simulink model "ABFTSMC"  (R2021b)
settings: Solver=VariableStepAuto  StartTime=0.0  StopTime=70  RelTol=1e-3
values from neighbouring files (symbols this model uses):
  a1 = (Iyy-Izz)/Ixx    [ABFTSMC_script.m]    (also in parameters_ABFTSMC.m = -1.00067938333)
  a10 = -kdy/m    [ABFTSMC_script.m]    (also in parameters_ABFTSMC.m = -0.00114547325103)
  a11 = -kdz/m    [ABFTSMC_script.m]    (also in parameters_ABFTSMC.m = -0.00114547325103)
  a3 = -kax/Ixx    [ABFTSMC_script.m]    (also in parameters_ABFTSMC.m = -0.145466422785)
  a4 = (Izz-Ixx)/Iyy    [ABFTSMC_script.m]    (also in parameters_ABFTSMC.m = 1.00067938333)
  a6 = -kay/Iyy    [ABFTSMC_script.m]    (also in parameters_ABFTSMC.m = -0.145466422785)
  a7 = (Ixx-Iyy)/Izz    [ABFTSMC_script.m]    (also in parameters_ABFTSMC.m = 0)
  a8 = -kaz/Izz    [ABFTSMC_script.m]    (also in parameters_ABFTSMC.m = -0.072708512917)
  a9 = -kdx/m    [ABFTSMC_script.m]    (also in parameters_ABFTSMC.m = -0.00114547325103)
  alpha_phi = 10    [ABFTSMC_script.m]    (also in parameters_ABFTSMC.m = 9.3414)
  alpha_si = 9.3414    [parameters_ABFTSMC.m]
  alpha_theta = alpha_phi    (= 10)    [ABFTSMC_script.m]    (also in parameters_ABFTSMC.m = 9.3414)
  b1 = 1/Ixx    [ABFTSMC_script.m]    (also in parameters_ABFTSMC.m = 39.1951920564)
  b2 = 1/Iyy    [ABFTSMC_script.m]    (also in parameters_ABFTSMC.m = 39.1951920564)
  b3 = 1/Izz    [ABFTSMC_script.m]    (also in parameters_ABFTSMC.m = 130.606274325)
  beta_phi = 0.2146    [ABFTSMC_script.m]    (also in parameters_ABFTSMC.m)
  beta_si = 0.2146    [parameters_ABFTSMC.m]
  beta_theta = beta_phi    (= 0.2146)    [ABFTSMC_script.m]    (also in parameters_ABFTSMC.m)
  c_phi = 0.01    [ABFTSMC_script.m]    (also in parameters_ABFTSMC.m = 0.0527)
  c_si = 0.0527    [parameters_ABFTSMC.m]
  c_theta = c_phi    (= 0.01)    [ABFTSMC_script.m]    (also in parameters_ABFTSMC.m = 0.0527)
  cd = Parameters.cd    [ABFTSMC_script.m]    (also in parameters_ABFTSMC.m = 0.03232)
  cx1 = 0.8    [ABFTSMC_script.m]    (also in parameters_ABFTSMC.m = 3.227)
  cy1 = 4    [ABFTSMC_script.m]    (also in parameters_ABFTSMC.m = 3.227)
  cz1 = 5    [ABFTSMC_script.m]    (also in parameters_ABFTSMC.m = 3.227)
  g = Parameters.g    [ABFTSMC_script.m]    (also in parameters_ABFTSMC.m = 9.81)
  gama11 = 0.1    [parameters_ABFTSMC.m]
  gama7 = 0.1    [parameters_ABFTSMC.m]
  gama9 = 0.1    [parameters_ABFTSMC.m]
  gama_phi = 17.4513    [parameters_ABFTSMC.m]
  gama_si = 17.4513    [parameters_ABFTSMC.m]
  gama_theta = 17.4513    [parameters_ABFTSMC.m]
  Ir = Parameters.Ir    [ABFTSMC_script.m]    (also in parameters_ABFTSMC.m = 2.8385e-05)
  Ixx = Parameters.Ixx    [ABFTSMC_script.m]    (also in parameters_ABFTSMC.m = 0.003827)
  Iyy = Parameters.Iyy    [ABFTSMC_script.m]    (also in parameters_ABFTSMC.m = 0.003827)
  kp = Parameters.kp    [ABFTSMC_script.m]    (also in parameters_ABFTSMC.m = 0.0029842)
  m = Parameters.m    [ABFTSMC_script.m]    (also in parameters_ABFTSMC.m = 0.486)
  mu = [mu_phi mu_theta mu_say]'    [ABFTSMC_script.m]    (also in parameters_ABFTSMC.m = 0.01*ones(3,1))
  p_phi = 3    [ABFTSMC_script.m]    (also in parameters_ABFTSMC.m = 2.4429)
  p_si = 2.4429    [parameters_ABFTSMC.m]
  p_theta = p_phi    (= 3)    [ABFTSMC_script.m]    (also in parameters_ABFTSMC.m = 2.4429)
  q_phi = 5    [ABFTSMC_script.m]    (also in parameters_ABFTSMC.m = 4.3864)
  q_si = 4.3864    [parameters_ABFTSMC.m]
  q_theta = q_phi    (= 5)    [ABFTSMC_script.m]    (also in parameters_ABFTSMC.m = 4.3864)
undefined symbols (not defined in the file or in its folder): magnitude
libraries: dspinverses x1
settings Model: Creator=alikh  LastModifiedBy=alikh

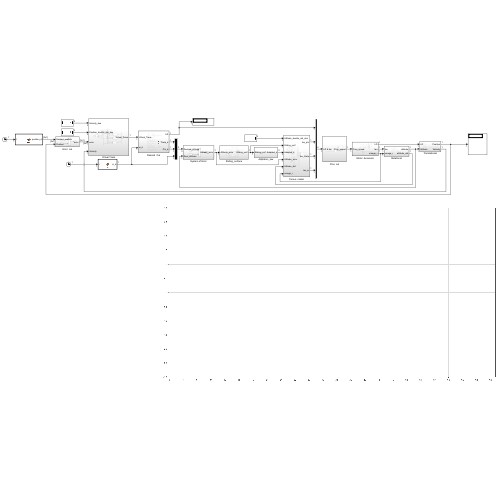
[thumbnail: Simulink's stored preview of the top-level diagram]
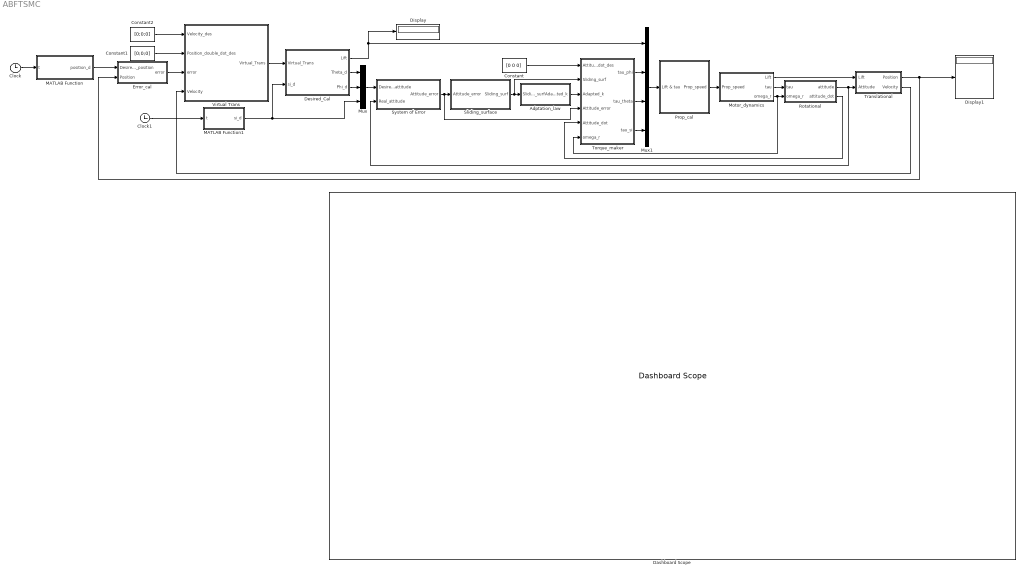
== system ABFTSMC ==
  Adptation_law : Subsystem
  Clock : Clock
  Clock1 : Clock
  Constant : Constant  Value=[0 0 0]
  Constant1 : Constant  Value=[0;0;0]
  Constant2 : Constant  Value=[0;0;0]
  Dashboard Scope : DashboardScope
  Desired_Cal : Subsystem
  Display : Display
  Display1 : Display
  Error_cal : Subsystem
  MATLAB Function : MATLAB Function  TreatAsAtomicUnit=on
  MATLAB Function1 : MATLAB Function  TreatAsAtomicUnit=on
  Motor_dynamics : Subsystem
  Mux : Mux  Inputs=3
  Mux1 : Mux
  Prop_cal : Subsystem
  Rotational : Subsystem
  Sliding_surface : Subsystem
  System of Error : Subsystem
  Torque_maker : Subsystem
  Translational : Subsystem
  Virtual Trans : Subsystem
  wires:
  Virtual Trans/1(Virtual_Trans) -> Desired_Cal/1(Virtual_Trans)
  MATLAB Function1/1(si_d) -> Desired_Cal/2(si_d), Mux/3
  Desired_Cal/2(Theta_d) -> Mux/1
  Desired_Cal/3(Phi_d) -> Mux/2
  Mux/1 -> System of Error/1(Desired_attitude)
  Desired_Cal/1(Lift) -> Display/1, Mux1/1
  System of Error/1(Attitude_error) -> Sliding_surface/1(Attitude_error), Torque_maker/4(Attitude_error)
  Sliding_surface/1(Sliding_surf) -> Torque_maker/2(Sliding_surf), Adptation_law/1(Sliding_surf)
  Adptation_law/1(Adapted_k) -> Torque_maker/3(Adapted_k)
  Torque_maker/1(tau_phi) -> Mux1/2
  Torque_maker/2(tau_theta) -> Mux1/3
  Torque_maker/3(tau_si) -> Mux1/4
  Mux1/1 -> Prop_cal/1(Lift & tau)
  Prop_cal/1(Prop_speed) -> Motor_dynamics/1(Prop_speed)
  Motor_dynamics/1(Lift) -> Translational/1(Lift)
  Motor_dynamics/2(tau) -> Rotational/1(tau)
  Motor_dynamics/3(omega_r) -> Torque_maker/6(omega_r), Rotational/2(omega_r)
  Rotational/2(attitude_dot) -> Torque_maker/5(Attitude_dot)
  Rotational/1(attitude) -> System of Error/2(Real_attitude), Translational/2(Attitude)
  Translational/2(Velocity) -> Virtual Trans/4(Velocity)
  Translational/1(Position) -> Error_cal/2(Position), Display1/1
  Error_cal/1(error) -> Virtual Trans/3(error)
  Constant/1 -> Torque_maker/1(Attitude_double_dot_des)
  Constant1/1 -> Virtual Trans/2(Position_double_dot_des)
  MATLAB Function/1(position_d) -> Error_cal/1(Desired_position)
  Clock/1 -> MATLAB Function/1(t)
  Clock1/1 -> MATLAB Function1/1(t)
  Constant2/1 -> Virtual Trans/1(Velocity_des)

== system ABFTSMC/Adptation_law ==
  Sliding_surf : Inport
  Abs : Abs
  Gain : Gain  Gain=[gama_phi gama_theta gama_si]'
  Integrator : Integrator
  Adapted_k : Outport
  wires:
  Gain/1 -> Integrator/1
  Sliding_surf/1 -> Abs/1
  Integrator/1 -> Adapted_k/1
  Abs/1 -> Gain/1

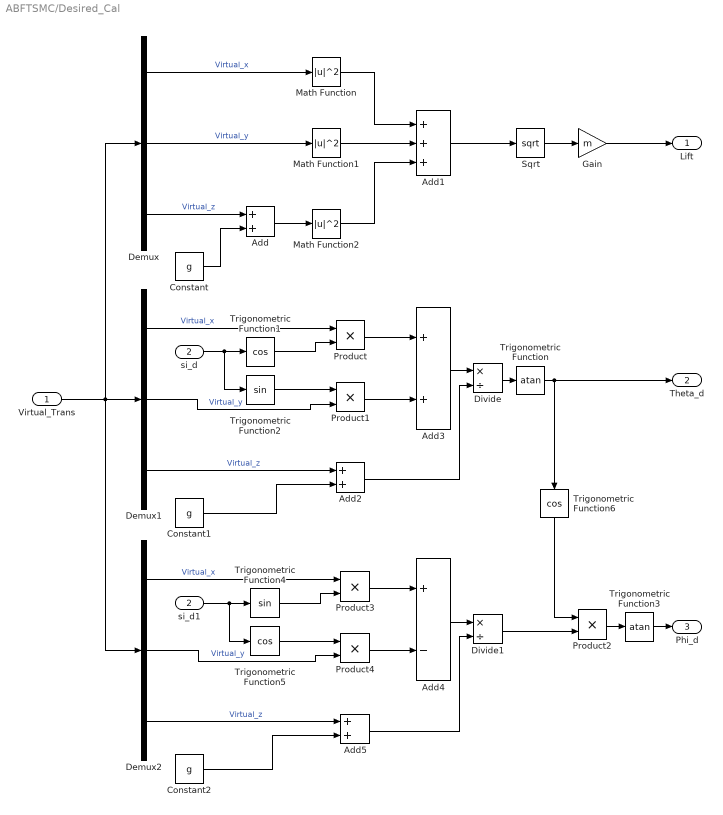
== system ABFTSMC/Desired_Cal ==
  Virtual_Trans : Inport
  si_d : Inport  Port=2
  Add{,2..3,5} (4 alike) : Sum
  Add1 : Sum  Inputs=+++
  Add4 : Sum  Inputs=+-
  Constant : Constant  Value=g
  Constant1 : Constant  Value=g
  Constant2 : Constant  Value=g
  Demux : Demux  Outputs=3
  Demux1 : Demux  Outputs=3
  Demux2 : Demux  Outputs=3
  Divide : Product  Inputs=*/
  Divide1 : Product  Inputs=*/
  Gain : Gain  Gain=m
  Math Function : Math  Operator=magnitude^2  SaturateOnIntegerOverflow=on
  Math Function1 : Math  Operator=magnitude^2  SaturateOnIntegerOverflow=on
  Math Function2 : Math  Operator=magnitude^2  SaturateOnIntegerOverflow=on
  Product{,1..4} (5 alike) : Product
  Sqrt : Sqrt  SaturateOnIntegerOverflow=on
  Trigonometric Function : Trigonometry  Operator=atan
  Trigonometric Function1 : Trigonometry  Operator=cos
  Trigonometric Function2 : Trigonometry
  Trigonometric Function3 : Trigonometry  Operator=atan
  Trigonometric Function4 : Trigonometry
  Trigonometric Function5 : Trigonometry  Operator=cos
  Trigonometric Function6 : Trigonometry  Operator=cos
  si_d1 : InportShadow  Port=2
  Lift : Outport
  Theta_d : Outport  Port=2
  Phi_d : Outport  Port=3
  wires:
  Virtual_Trans/1 -> Demux/1, Demux1/1, Demux2/1
  Demux/1 -> Math Function/1  "Virtual_x"
  Demux/2 -> Math Function1/1  "Virtual_y"
  Demux/3 -> Add/1  "Virtual_z"
  Constant/1 -> Add/2
  Add/1 -> Math Function2/1
  Add1/1 -> Sqrt/1
  Math Function1/1 -> Add1/2
  Sqrt/1 -> Gain/1
  Gain/1 -> Lift/1
  Math Function/1 -> Add1/1
  Math Function2/1 -> Add1/3
  si_d/1 -> Trigonometric Function2/1, Trigonometric Function1/1
  Demux1/1 -> Product/1  "Virtual_x"
  Trigonometric Function1/1 -> Product/2
  Trigonometric Function2/1 -> Product1/1
  Demux1/2 -> Product1/2  "Virtual_y"
  Demux1/3 -> Add2/1  "Virtual_z"
  Constant1/1 -> Add2/2
  Product/1 -> Add3/1
  Product1/1 -> Add3/2
  Add3/1 -> Divide/1
  Divide/1 -> Trigonometric Function/1
  Add2/1 -> Divide/2
  Trigonometric Function/1 -> Theta_d/1, Trigonometric Function6/1
  Trigonometric Function3/1 -> Phi_d/1
  Product2/1 -> Trigonometric Function3/1
  Add4/1 -> Divide1/1
  Product4/1 -> Add4/2
  Product3/1 -> Add4/1
  Demux2/2 -> Product4/2  "Virtual_y"
  Trigonometric Function5/1 -> Product4/1
  Trigonometric Function4/1 -> Product3/2
  Demux2/1 -> Product3/1  "Virtual_x"
  si_d1/1 -> Trigonometric Function4/1, Trigonometric Function5/1
  Demux2/3 -> Add5/1  "Virtual_z"
  Constant2/1 -> Add5/2
  Add5/1 -> Divide1/2
  Trigonometric Function6/1 -> Product2/1
  Divide1/1 -> Product2/2

== system ABFTSMC/Error_cal ==
  Desired_position : Inport
  Position : Inport  Port=2
  Add : Sum  Inputs=+-
  error : Outport
  wires:
  Position/1 -> Add/1
  Desired_position/1 -> Add/2
  Add/1 -> error/1

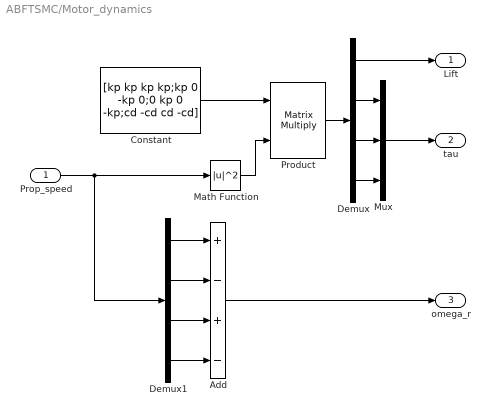
== system ABFTSMC/Motor_dynamics ==
  Prop_speed : Inport
  Add : Sum  Inputs=+-+-
  Constant : Constant  Value=[kp kp kp kp;kp 0 -kp 0;0 kp 0 -kp;cd -cd cd -cd]
  Demux : Demux
  Demux1 : Demux
  Math Function : Math  Operator=magnitude^2  SaturateOnIntegerOverflow=on
  Mux : Mux  Inputs=3
  Product : Product  Multiplication=Matrix(*)
  Lift : Outport
  tau : Outport  Port=2
  omega_r : Outport  Port=3
  wires:
  Constant/1 -> Product/1
  Math Function/1 -> Product/2
  Product/1 -> Demux/1
  Demux/1 -> Lift/1
  Demux/2 -> Mux/1
  Demux/3 -> Mux/2
  Demux/4 -> Mux/3
  Mux/1 -> tau/1
  Prop_speed/1 -> Math Function/1, Demux1/1
  Demux1/1 -> Add/1
  Demux1/2 -> Add/2
  Demux1/3 -> Add/3
  Demux1/4 -> Add/4
  Add/1 -> omega_r/1

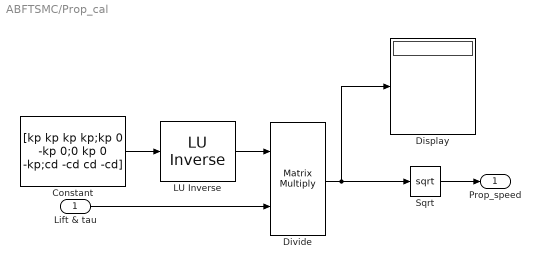
== system ABFTSMC/Prop_cal ==
  Lift & tau : Inport
  " LU Inverse" : dspinverses/ LU Inverse
  Constant : Constant  Value=[kp kp kp kp;kp 0 -kp 0;0 kp 0 -kp;cd -cd cd -cd]
  Display : Display
  Divide : Product  Inputs=**  Multiplication=Matrix(*)
  Sqrt : Sqrt  SaturateOnIntegerOverflow=on
  Prop_speed : Outport
  wires:
  Constant/1 -> " LU Inverse"/1
  Lift & tau/1 -> Divide/2
  " LU Inverse"/1 -> Divide/1
  Sqrt/1 -> Prop_speed/1
  Divide/1 -> Sqrt/1, Display/1

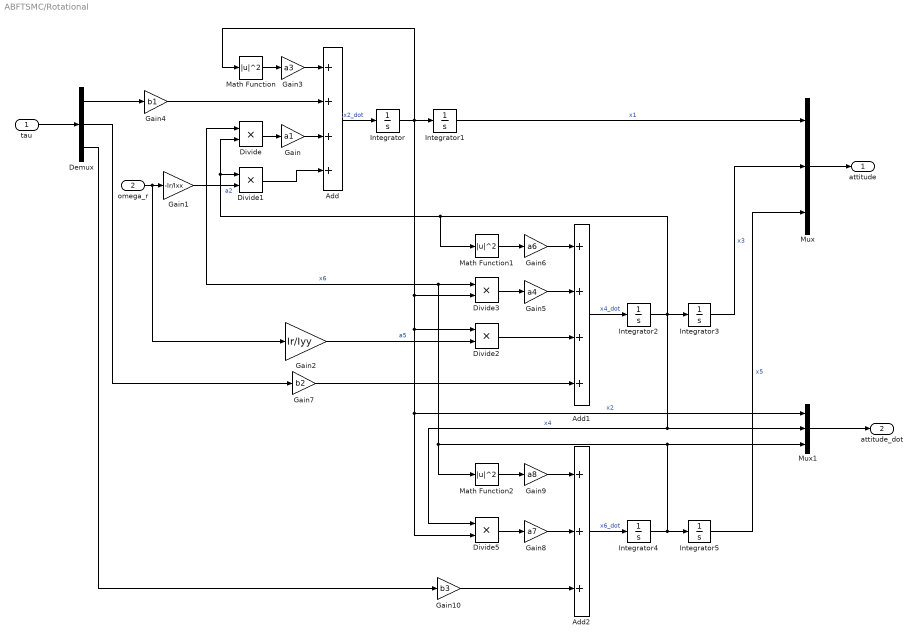
== system ABFTSMC/Rotational ==
  tau : Inport
  omega_r : Inport  Port=2
  Add : Sum  Inputs=++++
  Add1 : Sum  Inputs=++++
  Add2 : Sum  Inputs=+++
  Demux : Demux  Outputs=3
  Divide{,1..3,5} (5 alike) : Product  Inputs=**
  Gain : Gain  Gain=a1
  Gain1 : Gain  Gain=-Ir/Ixx
  Gain10 : Gain  Gain=b3
  Gain2 : Gain  Gain=Ir/Iyy
  Gain3 : Gain  Gain=a3
  Gain4 : Gain  Gain=b1
  Gain5 : Gain  Gain=a4
  Gain6 : Gain  Gain=a6
  Gain7 : Gain  Gain=b2
  Gain8 : Gain  Gain=a7
  Gain9 : Gain  Gain=a8
  Integrator{,1..5} (6 alike) : Integrator
  Math Function : Math  Operator=magnitude^2  SaturateOnIntegerOverflow=on
  Math Function1 : Math  Operator=magnitude^2  SaturateOnIntegerOverflow=on
  Math Function2 : Math  Operator=magnitude^2  SaturateOnIntegerOverflow=on
  Mux : Mux  Inputs=3
  Mux1 : Mux  Inputs=3
  attitude : Outport
  attitude_dot : Outport  Port=2
  wires:
  Divide/1 -> Gain/1
  Gain/1 -> Add/3
  omega_r/1 -> Gain2/1, Gain1/1
  Gain1/1 -> Divide1/2  "a2"
  Gain2/1 -> Divide2/2  "a5"
  Divide1/1 -> Add/4
  Math Function/1 -> Gain3/1
  tau/1 -> Demux/1
  Demux/1 -> Gain4/1
  Gain4/1 -> Add/2
  Add/1 -> Integrator/1  "x2_dot"
  Integrator/1 -> Integrator1/1, Divide3/2, Divide5/2, Mux1/1, Divide2/1, Math Function/1  "x2"
  Integrator1/1 -> Mux/1  "x1"
  Gain3/1 -> Add/1
  Mux/1 -> attitude/1
  Gain6/1 -> Add1/1
  Integrator3/1 -> Mux/2  "x3"
  Integrator2/1 -> Math Function1/1, Divide1/1, Divide/2, Integrator3/1, Divide5/1, Mux1/2  "x4"
  Add1/1 -> Integrator2/1  "x4_dot"
  Gain7/1 -> Add1/4
  Math Function1/1 -> Gain6/1
  Gain5/1 -> Add1/2
  Divide3/1 -> Gain5/1
  Demux/2 -> Gain7/1
  Divide2/1 -> Add1/3
  Divide5/1 -> Gain8/1
  Gain8/1 -> Add2/2
  Math Function2/1 -> Gain9/1
  Gain10/1 -> Add2/3
  Add2/1 -> Integrator4/1  "x6_dot"
  Integrator4/1 -> Integrator5/1, Divide3/1, Divide/1, Math Function2/1, Mux1/3  "x6"
  Integrator5/1 -> Mux/3  "x5"
  Gain9/1 -> Add2/1
  Demux/3 -> Gain10/1
  Mux1/1 -> attitude_dot/1

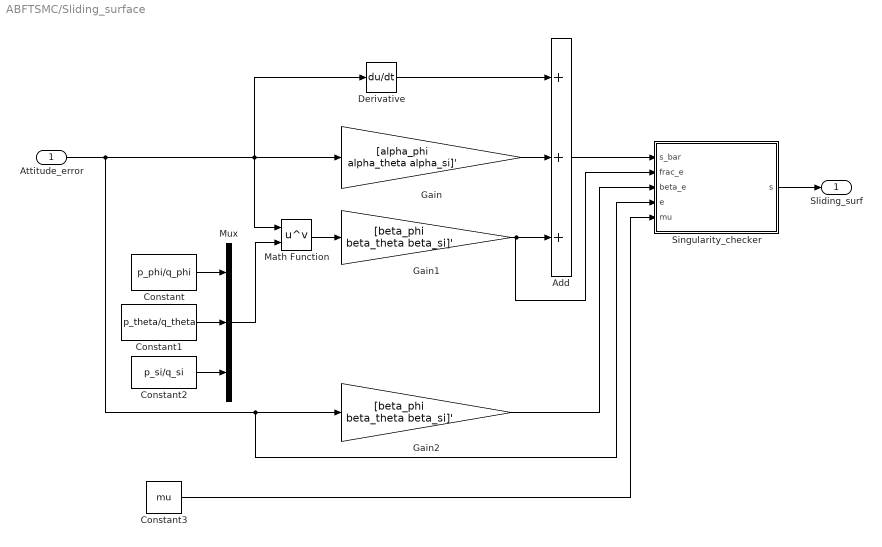
== system ABFTSMC/Sliding_surface ==
  Attitude_error : Inport
  Add : Sum  Inputs=+++
  Constant : Constant  Value=p_phi/q_phi
  Constant1 : Constant  Value=p_theta/q_theta
  Constant2 : Constant  Value=p_si/q_si
  Constant3 : Constant  Value=mu
  Derivative : Derivative
  Gain : Gain  Gain=[alpha_phi alpha_theta alpha_si]'
  Gain1 : Gain  Gain=[beta_phi beta_theta beta_si]'
  Gain2 : Gain  Gain=[beta_phi beta_theta beta_si]'
  Math Function : Math  Operator=pow  SaturateOnIntegerOverflow=on
  Mux : Mux  Inputs=3
  Singularity_checker : MATLAB Function  TreatAsAtomicUnit=on
  Sliding_surf : Outport
  wires:
  Attitude_error/1 -> Derivative/1, Math Function/1, Gain/1, Gain2/1, Singularity_checker/4(e)
  Derivative/1 -> Add/1
  Gain/1 -> Add/2
  Gain1/1 -> Singularity_checker/2(frac_e), Add/3
  Math Function/1 -> Gain1/1
  Constant/1 -> Mux/1
  Constant1/1 -> Mux/2
  Constant2/1 -> Mux/3
  Mux/1 -> Math Function/2
  Add/1 -> Singularity_checker/1(s_bar)
  Gain2/1 -> Singularity_checker/3(beta_e)
  Singularity_checker/1(s) -> Sliding_surf/1
  Constant3/1 -> Singularity_checker/5(mu)

== system ABFTSMC/System of Error ==
  Desired_attitude : Inport
  Real_attitude : Inport  Port=2
  Add : Sum  Inputs=+-
  Attitude_error : Outport
  wires:
  Real_attitude/1 -> Add/1
  Desired_attitude/1 -> Add/2
  Add/1 -> Attitude_error/1

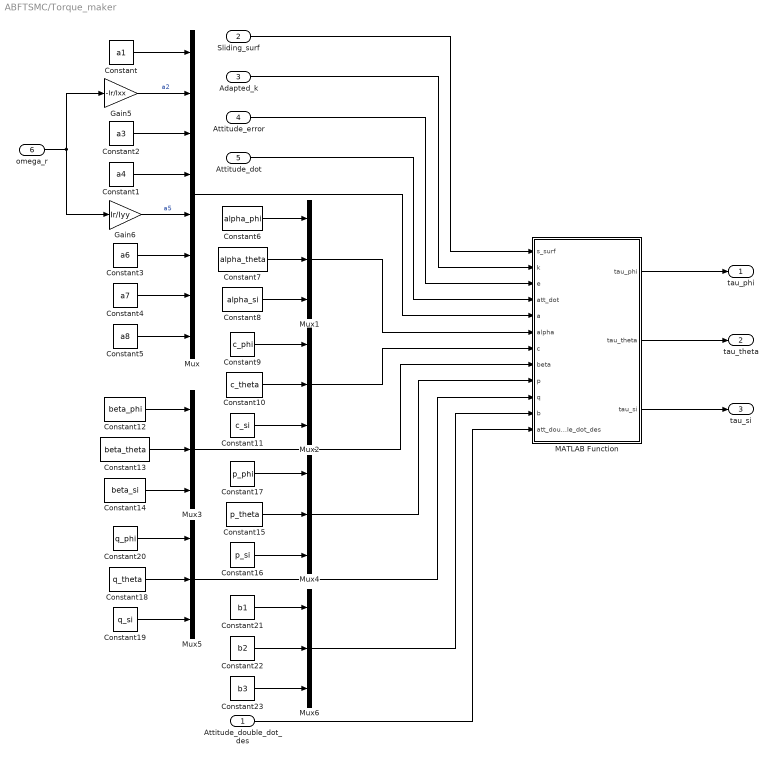
== system ABFTSMC/Torque_maker ==
  Attitude_double_dot_des : Inport
  Sliding_surf : Inport  Port=2
  Adapted_k : Inport  Port=3
  Attitude_error : Inport  Port=4
  Attitude_dot : Inport  Port=5
  omega_r : Inport  Port=6
  Constant : Constant  Value=a1
  Constant1 : Constant  Value=a4
  Constant10 : Constant  Value=c_theta
  Constant11 : Constant  Value=c_si
  Constant12 : Constant  Value=beta_phi
  Constant13 : Constant  Value=beta_theta
  Constant14 : Constant  Value=beta_si
  Constant15 : Constant  Value=p_theta
  Constant16 : Constant  Value=p_si
  Constant17 : Constant  Value=p_phi
  Constant18 : Constant  Value=q_theta
  Constant19 : Constant  Value=q_si
  Constant2 : Constant  Value=a3
  Constant20 : Constant  Value=q_phi
  Constant21 : Constant  Value=b1
  Constant22 : Constant  Value=b2
  Constant23 : Constant  Value=b3
  Constant3 : Constant  Value=a6
  Constant4 : Constant  Value=a7
  Constant5 : Constant  Value=a8
  Constant6 : Constant  Value=alpha_phi
  Constant7 : Constant  Value=alpha_theta
  Constant8 : Constant  Value=alpha_si
  Constant9 : Constant  Value=c_phi
  Gain5 : Gain  Gain=-Ir/Ixx
  Gain6 : Gain  Gain=Ir/Iyy
  MATLAB Function : MATLAB Function  TreatAsAtomicUnit=on
  Mux : Mux  Inputs=8
  Mux{1..6} (6 alike) : Mux  Inputs=3
  tau_phi : Outport
  tau_theta : Outport  Port=2
  tau_si : Outport  Port=3
  wires:
  Gain5/1 -> Mux/2  "a2"
  omega_r/1 -> Gain5/1, Gain6/1
  Constant/1 -> Mux/1
  Constant2/1 -> Mux/3
  Constant1/1 -> Mux/4
  Gain6/1 -> Mux/5  "a5"
  Constant3/1 -> Mux/6
  Constant4/1 -> Mux/7
  Constant5/1 -> Mux/8
  Constant6/1 -> Mux1/1
  Constant7/1 -> Mux1/2
  Constant8/1 -> Mux1/3
  Constant9/1 -> Mux2/1
  Constant10/1 -> Mux2/2
  Constant11/1 -> Mux2/3
  Constant14/1 -> Mux3/3
  Constant13/1 -> Mux3/2
  Constant12/1 -> Mux3/1
  Constant16/1 -> Mux4/3
  Constant15/1 -> Mux4/2
  Constant17/1 -> Mux4/1
  Constant20/1 -> Mux5/1
  Constant18/1 -> Mux5/2
  Constant19/1 -> Mux5/3
  Sliding_surf/1 -> MATLAB Function/1(s_surf)
  Adapted_k/1 -> MATLAB Function/2(k)
  Attitude_error/1 -> MATLAB Function/3(e)
  Attitude_dot/1 -> MATLAB Function/4(att_dot)
  Mux/1 -> MATLAB Function/5(a)
  Mux1/1 -> MATLAB Function/6(alpha)
  Mux2/1 -> MATLAB Function/7(c)
  Mux3/1 -> MATLAB Function/8(beta)
  Mux4/1 -> MATLAB Function/9(p)
  Mux5/1 -> MATLAB Function/10(q)
  MATLAB Function/3(tau_si) -> tau_si/1
  MATLAB Function/2(tau_theta) -> tau_theta/1
  MATLAB Function/1(tau_phi) -> tau_phi/1
  Constant23/1 -> Mux6/3
  Constant22/1 -> Mux6/2
  Constant21/1 -> Mux6/1
  Mux6/1 -> MATLAB Function/11(b)
  Attitude_double_dot_des/1 -> MATLAB Function/12(att_double_dot_des)

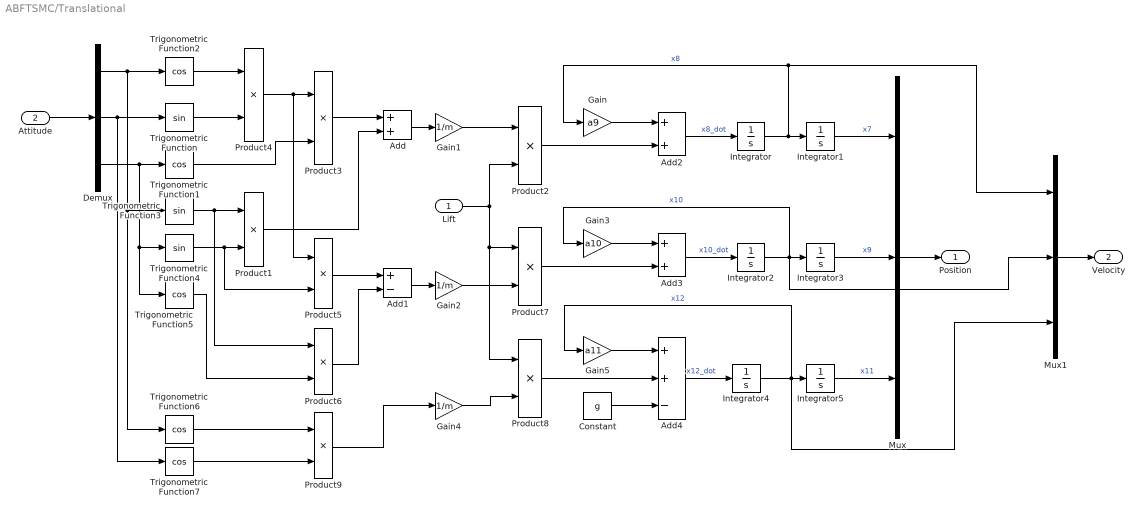
== system ABFTSMC/Translational ==
  Lift : Inport
  Attitude : Inport  Port=2
  Add : Sum
  Add1 : Sum  Inputs=+-
  Add2 : Sum
  Add3 : Sum
  Add4 : Sum  Inputs=++-
  Constant : Constant  Value=g
  Demux : Demux  Outputs=3
  Gain : Gain  Gain=a9
  Gain1 : Gain  Gain=1/m
  Gain2 : Gain  Gain=1/m
  Gain3 : Gain  Gain=a10
  Gain4 : Gain  Gain=1/m
  Gain5 : Gain  Gain=a11
  Integrator{,1..5} (6 alike) : Integrator
  Mux : Mux  Inputs=3
  Mux1 : Mux  Inputs=3
  Product{1..9} (9 alike) : Product
  Trigonometric Function : Trigonometry
  Trigonometric Function{1..2,5..7} (5 alike) : Trigonometry  Operator=cos
  Trigonometric Function3 : Trigonometry
  Trigonometric Function4 : Trigonometry
  Position : Outport
  Velocity : Outport  Port=2
  wires:
  Attitude/1 -> Demux/1
  Demux/1 -> Trigonometric Function2/1, Trigonometric Function6/1, Trigonometric Function3/1
  Demux/2 -> Trigonometric Function7/1, Trigonometric Function/1
  Demux/3 -> Trigonometric Function1/1, Trigonometric Function4/1, Trigonometric Function5/1
  Trigonometric Function2/1 -> Product4/1
  Trigonometric Function/1 -> Product4/2
  Trigonometric Function4/1 -> Product1/2, Product5/2
  Trigonometric Function3/1 -> Product1/1, Product6/1
  Product1/1 -> Add/2
  Add/1 -> Gain1/1
  Lift/1 -> Product8/1, Product7/1, Product2/2
  Gain1/1 -> Product2/1
  Product4/1 -> Product3/1, Product5/1
  Trigonometric Function1/1 -> Product3/2
  Product3/1 -> Add/1
  Product5/1 -> Add1/1
  Product6/1 -> Add1/2
  Trigonometric Function5/1 -> Product6/2
  Add1/1 -> Gain2/1
  Gain2/1 -> Product7/2
  Add2/1 -> Integrator/1  "x8_dot"
  Integrator/1 -> Mux1/1, Gain/1, Integrator1/1  "x8"
  Gain/1 -> Add2/1
  Integrator1/1 -> Mux/1  "x7"
  Product2/1 -> Add2/2
  Product7/1 -> Add3/2
  Add3/1 -> Integrator2/1  "x10_dot"
  Integrator2/1 -> Mux1/2, Gain3/1, Integrator3/1  "x10"
  Integrator3/1 -> Mux/2  "x9"
  Gain3/1 -> Add3/1
  Mux/1 -> Position/1
  Gain4/1 -> Product8/2
  Trigonometric Function6/1 -> Product9/1
  Trigonometric Function7/1 -> Product9/2
  Product9/1 -> Gain4/1
  Integrator5/1 -> Mux/3  "x11"
  Integrator4/1 -> Mux1/3, Gain5/1, Integrator5/1  "x12"
  Add4/1 -> Integrator4/1  "x12_dot"
  Gain5/1 -> Add4/1
  Product8/1 -> Add4/2
  Constant/1 -> Add4/3
  Mux1/1 -> Velocity/1

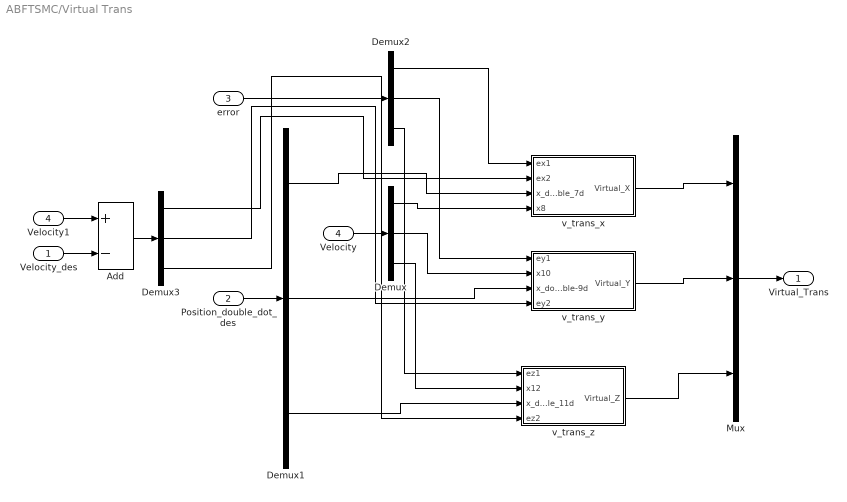
== system ABFTSMC/Virtual Trans ==
  Velocity_des : Inport
  Position_double_dot_des : Inport  Port=2
  error : Inport  Port=3
  Velocity : Inport  Port=4
  Add : Sum  Inputs=+-
  Demux{,1..3} (4 alike) : Demux  Outputs=3
  Mux : Mux  Inputs=3
  Velocity1 : InportShadow  Port=4
  v_trans_x : Subsystem
  v_trans_y : Subsystem
  v_trans_z : Subsystem
  Virtual_Trans : Outport
  wires:
  Demux/1 -> v_trans_x/4(x8)
  Demux/2 -> v_trans_y/2(x10)
  Demux/3 -> v_trans_z/2(x12)
  Mux/1 -> Virtual_Trans/1
  v_trans_y/1(Virtual_Y) -> Mux/2
  v_trans_x/1(Virtual_X) -> Mux/1
  v_trans_z/1(Virtual_Z) -> Mux/3
  Velocity/1 -> Demux/1
  Position_double_dot_des/1 -> Demux1/1
  Demux1/1 -> v_trans_x/3(x_double_7d)
  Demux1/2 -> v_trans_y/3(x_double-9d)
  Demux1/3 -> v_trans_z/3(x_double_11d)
  error/1 -> Demux2/1
  Demux2/1 -> v_trans_x/1(ex1)
  Demux2/2 -> v_trans_y/1(ey1)
  Demux2/3 -> v_trans_z/1(ez1)
  Velocity1/1 -> Add/1
  Velocity_des/1 -> Add/2
  Add/1 -> Demux3/1
  Demux3/1 -> v_trans_x/2(ex2)
  Demux3/2 -> v_trans_y/4(ey2)
  Demux3/3 -> v_trans_z/4(ez2)

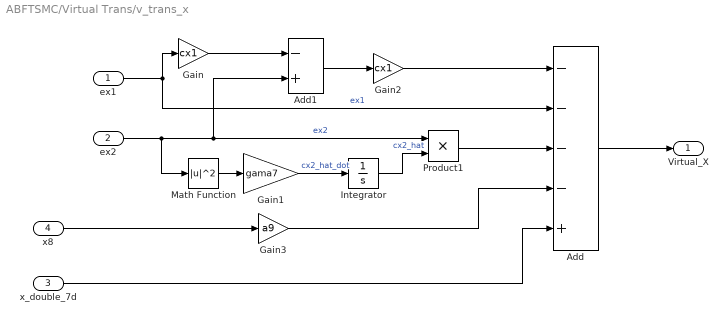
== system ABFTSMC/Virtual Trans/v_trans_x ==
  ex1 : Inport
  ex2 : Inport  Port=2
  x_double_7d : Inport  Port=3
  x8 : Inport  Port=4
  Add : Sum  Inputs=----+
  Add1 : Sum  Inputs=-+
  Gain : Gain  Gain=cx1
  Gain1 : Gain  Gain=gama7
  Gain2 : Gain  Gain=cx1
  Gain3 : Gain  Gain=a9
  Integrator : Integrator
  Math Function : Math  Operator=magnitude^2  SaturateOnIntegerOverflow=on
  Product1 : Product
  Virtual_X : Outport
  wires:
  ex2/1 -> Math Function/1, Add1/2, Product1/1  "ex2"
  Math Function/1 -> Gain1/1
  Add/1 -> Virtual_X/1
  ex1/1 -> Add/2, Gain/1  "ex1"
  Gain1/1 -> Integrator/1  "cx2_hat_dot"
  Integrator/1 -> Product1/2  "cx2_hat"
  Product1/1 -> Add/3
  Gain/1 -> Add1/1
  Add1/1 -> Gain2/1
  Gain2/1 -> Add/1
  x8/1 -> Gain3/1
  Gain3/1 -> Add/4
  x_double_7d/1 -> Add/5

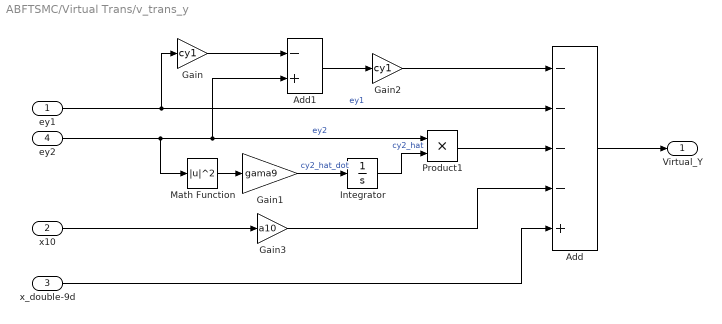
== system ABFTSMC/Virtual Trans/v_trans_y ==
  ey1 : Inport
  x10 : Inport  Port=2
  x_double-9d : Inport  Port=3
  ey2 : Inport  Port=4
  Add : Sum  Inputs=----+
  Add1 : Sum  Inputs=-+
  Gain : Gain  Gain=cy1
  Gain1 : Gain  Gain=gama9
  Gain2 : Gain  Gain=cy1
  Gain3 : Gain  Gain=a10
  Integrator : Integrator
  Math Function : Math  Operator=magnitude^2  SaturateOnIntegerOverflow=on
  Product1 : Product
  Virtual_Y : Outport
  wires:
  Add/1 -> Virtual_Y/1
  Gain3/1 -> Add/4
  x_double-9d/1 -> Add/5
  ey2/1 -> Math Function/1, Add1/2, Product1/1  "ey2"
  Integrator/1 -> Product1/2  "cy2_hat"
  Gain1/1 -> Integrator/1  "cy2_hat_dot"
  Gain/1 -> Add1/1
  Math Function/1 -> Gain1/1
  ey1/1 -> Gain/1, Add/2  "ey1"
  x10/1 -> Gain3/1
  Add1/1 -> Gain2/1
  Gain2/1 -> Add/1
  Product1/1 -> Add/3

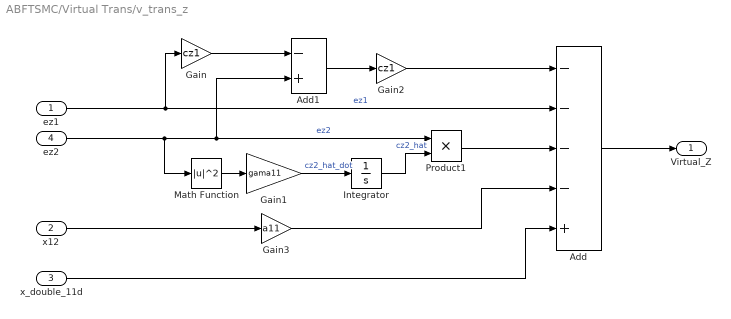
== system ABFTSMC/Virtual Trans/v_trans_z ==
  ez1 : Inport
  x12 : Inport  Port=2
  x_double_11d : Inport  Port=3
  ez2 : Inport  Port=4
  Add : Sum  Inputs=----+
  Add1 : Sum  Inputs=-+
  Gain : Gain  Gain=cz1
  Gain1 : Gain  Gain=gama11
  Gain2 : Gain  Gain=cz1
  Gain3 : Gain  Gain=a11
  Integrator : Integrator
  Math Function : Math  Operator=magnitude^2  SaturateOnIntegerOverflow=on
  Product1 : Product
  Virtual_Z : Outport
  wires:
  Add/1 -> Virtual_Z/1
  Gain3/1 -> Add/4
  x_double_11d/1 -> Add/5
  ez2/1 -> Math Function/1, Add1/2, Product1/1  "ez2"
  Integrator/1 -> Product1/2  "cz2_hat"
  Gain1/1 -> Integrator/1  "cz2_hat_dot"
  Gain/1 -> Add1/1
  Math Function/1 -> Gain1/1
  ez1/1 -> Gain/1, Add/2  "ez1"
  x12/1 -> Gain3/1
  Add1/1 -> Gain2/1
  Gain2/1 -> Add/1
  Product1/1 -> Add/3

== matlab function ABFTSMC/Torque_maker/MATLAB Function ==
  data: s_surf input; tau_phi output; k input; e input; att_dot input; a input; alpha input; c input; beta input; p input; q input; tau_theta output; tau_si output; b input; att_double_dot_des input
function [tau_phi,tau_theta,tau_si] = fcn(s_surf,k,e,att_dot,a,alpha,c,beta,p,q,b,att_double_dot_des)
s_phi=s_surf(1);s_theta=s_surf(2);s_si=s_surf(3);
k_phi=k(1);k_theta=k(2);k_si=k(3);
e_phi=e(1);e_theta=e(2);e_si=e(3);
x2=att_dot(1);x4=att_dot(2);x6=att_dot(3);
a1=a(1);a2=a(2);a3=a(3);a4=a(4);a5=a(5);
a6=a(6);a7=a(7);a8=a(8);
alpha_phi=alpha(1);alpha_theta=alpha(2);alpha_si=alpha(3);
c_phi=c(1);c_theta=c(2);c_si=c(3);
beta_phi=beta(1);beta_theta=beta(2);beta_si=beta(3);
p_phi=p(1);p_theta=p(2);p_si=p(3);
q_phi=q(1);q_theta=q(2);q_si=q(3);
b1=b(1);b2=b(2);b3=b(3);
xdd1=att_double_dot_des(1);xdd3=att_double_dot_des(2);
xdd5=att_double_dot_des(3);

tau_phi=1/b1*(-(a1*x4*x6+a2*x4+a3*x2^2)+xdd1-alpha_phi*(s_phi-c_phi*e_phi)+...
    p_phi/q_phi*beta_phi*e_phi^(p_phi/q_phi-1)-k_phi*sign(s_phi));

tau_theta=1/b2*(-(a4*x2*x6+a5*x2+a6*x4^2)+xdd3-alpha_theta*(s_theta-c_theta*e_theta)+...
    p_theta/q_theta*beta_theta*e_theta^(p_theta/q_theta-1)-k_theta*sign(s_theta));

tau_si=1/b3*(-(a7*x2*x4+a8*x6^2)+xdd5-alpha_si*(s_si-c_si*e_si)+...
    p_si/q_si*beta_si*e_si^(p_si/q_si-1)-k_si*sign(s_si));

== matlab function ABFTSMC/Sliding_surface/Singularity_checker ==
  data: s_bar input; s output; frac_e input; beta_e input; e input; mu input
function s = reviser(s_bar,frac_e,beta_e,e,mu)
s=zeros(3,1);
for i=1:3
if s_bar(i)~=0 & abs(e(i))<=mu(i)
s(i)=s_bar(i)-frac_e(i)+beta_e(i);
else
s(i)=s_bar(i);
end
end
end

== matlab function ABFTSMC/MATLAB Function ==
  data: t input; position_d output
function position_d = fcn(t)
position_d=zeros(3,1);
if t<10
    position_d=0.6*ones(3,1);
elseif t>=10 & t<20
    position_d=[0.3;0.6;0.6];
elseif t>=20 & t<30
    position_d=[0.3;0.3;0.6];
elseif t>=30 & t<40
    position_d=[0.6;0.3;0.6];
elseif t>=40 & t<50
    position_d=[0.6;0.6;0.6];
elseif t>=50
    position_d=[0.6;0.6;0];
end

== matlab function ABFTSMC/MATLAB Function1 ==
  data: t input; si_d output
function si_d = fcn(t)
if t<50
    si_d=0.5;
else
    si_d=0;
end
